simulink model "testing4"  (R2022a)
settings: Solver=VariableStepAuto  StartTime=0.0  StopTime=50  RelTol=1e-7
libraries: fuzblock x1
settings Model: Creator=mikol  LastModifiedBy=mikol

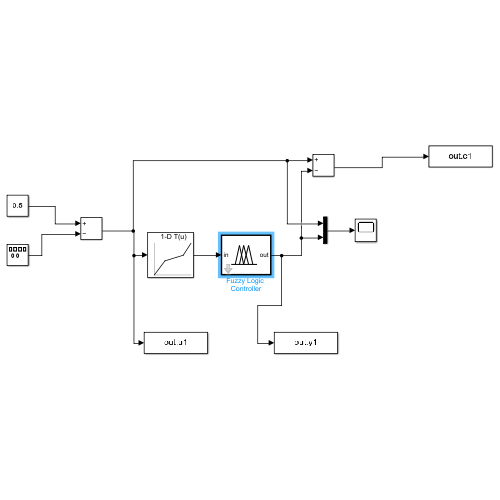
[thumbnail: Simulink's stored preview of the top-level diagram]
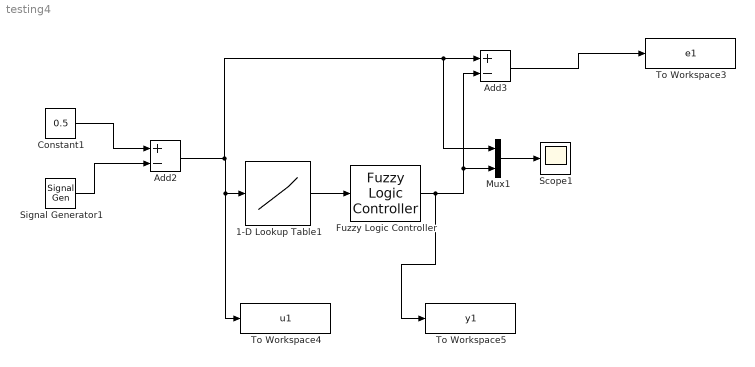
== system testing4 ==
  1-D Lookup Table1 : Lookup_n-D  NumberOfTableDimensions=1  BreakpointsForDimension1=[0 0.3 0.6 0.8 1]  Table=[3 7 8 8.5 12]  InternalRulePriority=Speed  RndMeth=Simplest
  Add2 : Sum  Inputs=+-
  Add3 : Sum  Inputs=+-
  Constant1 : Constant  Value=0.5
  Fuzzy Logic Controller : fuzblock/Fuzzy Logic  Controller  FIS=trimf2  OutputSampleNumber=101  DataType=double  FuzzifiedInputs=off  RuleFiringStrengths=off  RuleOutputs=off  AggregatedOutputs=off  SimulateUsing=Interpreted execution  OutOfRangeInputValueMessage=warning  NoRuleFiredMessage=warning  EmptyOutputFuzzySetMessage=warning
  Mux1 : Mux  Inputs=2
  Scope1 : Scope
  Signal Generator1 : SignalGenerator  Amplitude=0.5  Units=rad/sec
  To Workspace3 : ToWorkspace  VariableName=e1  SaveFormat=Timeseries  SampleTime=0.1
  To Workspace4 : ToWorkspace  VariableName=u1  SaveFormat=Timeseries  SampleTime=0.1
  To Workspace5 : ToWorkspace  VariableName=y1  SaveFormat=Timeseries  SampleTime=0.1
      settings: Save2DSignal=2-D array (concatenate along first dimension)
  wires:
  Add3/1 -> To Workspace3/1
  Add2/1 -> Mux1/1, Add3/1, To Workspace4/1, 1-D Lookup Table1/1
  Signal Generator1/1 -> Add2/2
  Mux1/1 -> Scope1/1
  Fuzzy Logic Controller/1 -> To Workspace5/1, Add3/2, Mux1/2
  1-D Lookup Table1/1 -> Fuzzy Logic Controller/1
  Constant1/1 -> Add2/1
